simulink model "DQN_ABC_Test"  (R2023b)
settings: Solver=ode23tb  StartTime=0.0  StopTime=0.1  FixedStep=Ts  RelTol=1e-3
values from neighbouring files (symbols this model uses):
  Carm = 3.76    [DQn_ABC_Test_calc.m]
  L = Ld + Lm    [DQn_ABC_Test_calc.m]
  La = 1e-3    (= 0.001)    [DQn_ABC_Test_calc.m]
  Lb = 2*La    (= 0.002)    [DQn_ABC_Test_calc.m]
  Lc = 0.5*La    (= 0.0005)    [DQn_ABC_Test_calc.m]
  N = 1    [DQn_ABC_Test_calc.m]
  R = Rd + Rm    [DQn_ABC_Test_calc.m]
  Ra = 1.64    [DQn_ABC_Test_calc.m]
  Rb = 1.4*Ra    (= 2.296)    [DQn_ABC_Test_calc.m]
  Rc = 2.8*Ra    (= 4.592)    [DQn_ABC_Test_calc.m]
  Ta_dqn = oDP.Ta_dqn    [DQn_ABC_Test_calc.m]
  Ts = 50e-6    (= 5e-05)    [DQn_ABC_Test_calc.m]
  Ts_dqn = Ts    (= 5e-05)    [DQn_ABC_Test_calc.m]
  Ts_emt = Ts    (= 5e-05)    [DQn_ABC_Test_calc.m]
  Ws = 2*pi*f    (= 314.159265359)    [DQn_ABC_Test_calc.m]
undefined symbols (not defined in the file or in its folder): DiscIntNeverNeededParam, i, Xdcpnz, Xdcpnz_c, Xpnz, Ydcpnz, Ydcpnz_c, Ypnz
libraries: DQN_Lib x81, spsCurrentMeasurementLib x9, spsControlledVoltageSourceLib x9, spsSeriesRLCBranchLib x6, spsGroundLib x6, simulink x3, spsMutualInductanceLib x1, spspowerguiLib x1
(part 3 of 6)

== matlab function DQN_ABC_Test/Mult_DQN_Mat4 ==
  data: Xdcpnz_c input; Ydcpnz_c input; Z_DQN output; N parameter; HrmDbl parameter; Zdcpnz_c output
function [Z_DQN, Zdcpnz_c]   = MultDQN(Xdcpnz_c, Ydcpnz_c, N, HrmDbl)

    X_DQN = zeros(N+1,6);
    Y_DQN = zeros(N+1,6);
    Z_DQN = zeros(2*N+1,6);
    Zdcpnz_c = complex(zeros(3,2*N+1));

    X_DQN(1,4) =  2*real(Xdcpnz_c(1,1));
    X_DQN(1,5) =  2*real(Xdcpnz_c(2,1));
    X_DQN(1,6) =  real(Xdcpnz_c(3,1));

    X_DQN(1,1) =  -2*imag(Xdcpnz_c(1,1));
    X_DQN(1,2) =  2*imag(Xdcpnz_c(2,1));
    X_DQN(1,3) =  imag(Xdcpnz_c(3,1));

    Y_DQN(1,4) =  2*real(Ydcpnz_c(1,1));
    Y_DQN(1,5) =  2*real(Ydcpnz_c(2,1));
    Y_DQN(1,6) =  real(Ydcpnz_c(3,1));

    Y_DQN(1,1) =  -2*imag(Ydcpnz_c(1,1));
    Y_DQN(1,2) =  2*imag(Ydcpnz_c(2,1));
    Y_DQN(1,3) =  imag(Ydcpnz_c(3,1));
    
    for i = 2 : N + 1
    
        X_DQN(i,1) =  real(Xdcpnz_c(1,i));
        X_DQN(i,2) = -real(Xdcpnz_c(2,i));
        X_DQN(i,3) =  real(Xdcpnz_c(3,i));

        X_DQN(i,4) =  imag(Xdcpnz_c(1,i));
        X_DQN(i,5) =  imag(Xdcpnz_c(2,i));
        X_DQN(i,6) =  imag(Xdcpnz_c(3,i));

        Y_DQN(i,1) =  real(Ydcpnz_c(1,i));
        Y_DQN(i,2) = -real(Ydcpnz_c(2,i));
        Y_DQN(i,3) =  real(Ydcpnz_c(3,i));

        Y_DQN(i,4) =  imag(Ydcpnz_c(1,i));
        Y_DQN(i,5) =  imag(Ydcpnz_c(2,i));
        Y_DQN(i,6) =  imag(Ydcpnz_c(3,i));
    
    end


%%%%%%%%%%%%%%%%%%%%%%%%%%%%%%

    Xdp = X_DQN(:,1);
    Xdn = X_DQN(:,2);
    Xdz = X_DQN(:,3);
    Xqp = X_DQN(:,4);
    Xqn = X_DQN(:,5);
    Xqz = X_DQN(:,6);
    
    Ydp = Y_DQN(:,1);
    Ydn = Y_DQN(:,2);
    Ydz = Y_DQN(:,3);
    Yqp = Y_DQN(:,4);
    Yqn = Y_DQN(:,5);
    Yqz = Y_DQN(:,6);
    
    Xdc = zeros(6,1);
    Ydc = zeros(6,1);
    Zdc = zeros(6,1);

    Xdc(1) = Xdp(1);
    Xdc(2) = Xdn(1);
    Xdc(3) = Xdz(1);
    Xdc(4) = Xqp(1);
    Xdc(5) = Xqn(1);
    Xdc(6) = Xqz(1);

    Ydc(1) = Ydp(1);
    Ydc(2) = Ydn(1);
    Ydc(3) = Ydz(1);
    Ydc(4) = Yqp(1);
    Ydc(5) = Yqn(1);
    Ydc(6) = Yqz(1);

    a = -0.5+0.866i;
    a2 = -0.5-0.866i;
    T = [1 1 1;1 a a2;1 a2 a];    

    Xdp = [Xdp(2:end); zeros(N-numel(Xdp)+1,1)];
    Ydp = [Ydp(2:end); zeros(N-numel(Ydp)+1,1)];
    Xqp = [Xqp(2:end); zeros(N-numel(Xqp)+1,1)];
    Yqp = [Yqp(2:end); zeros(N-numel(Yqp)+1,1)];
      
    Xdn = [Xdn(2:end); zeros(N-numel(Xdn)+1,1)];
    Ydn = [Ydn(2:end); zeros(N-numel(Ydn)+1,1)];
    Xqn = [Xqn(2:end); zeros(N-numel(Xqn)+1,1)];
    Yqn = [Yqn(2:end); zeros(N-numel(Yqn)+1,1)];
    
    Xdz = [Xdz(2:end); zeros(N-numel(Xdz)+1,1)];
    Ydz = [Ydz(2:end); zeros(N-numel(Ydz)+1,1)];
    Xqz = [Xqz(2:end); zeros(N-numel(Xqz)+1,1)];
    Yqz = [Yqz(2:end); zeros(N-numel(Yqz)+1,1)];
    
   

    Tad_p = [0      -sqrt(1/3)   sqrt(1/3);
            (2/3)   -(1/3)      -(1/3);
            (1/3)    (1/3)       (1/3)];

    Tda_p = [-0           1     1;
             -sqrt(3/4)  -0.5   1;
              sqrt(3/4)  -0.5   1;];


    Tdqn_a = [Tda_p(:,1)  Tda_p(:,1)  0*Tda_p(:,3)  Tda_p(:,2)  Tda_p(:,2)  2*Tda_p(:,3)]/2;
    Ta_dqn = [Tad_p(1,:); Tad_p(1,:); 0*Tad_p(3,:); Tad_p(2,:); Tad_p(2,:); Tad_p(3,:)];
    
    if(0)

        Zdc([1,4, 3]) = Tad_p*((Tda_p*Xdc([1,4,3])).*(Tda_p*Ydc([1,4,3])));
    
    else

        a = -0.5+0.866i;
        a2 = -0.5-0.866i;
        Sas = [1,a,a2;1,a2,a;1,1,1]/3;
        Ssa = inv(Sas);
       

        Zdc = Ta_dqn*((Tdqn_a*Xdc).*(Tdqn_a*Ydc));

    end
    
         
    %Zdc = Xdc.*Ydc;
       
    for h = 1 : 2*N
        if(h<=N)

            Zdc = Zdc + Ta_dqn*0.5*((Xdp(h)*Ydp(h)+Xqp(h)*Yqp(h)+Xdn(h)*Ydn(h)+Xqn(h)*Yqn(h)+Xdz(h)*Ydz(h)+Xqz(h)*Yqz(h))*[1;1;1]);

            %Zdc = Zdc + 0.5*real(Xdcpnz_c(:,h)'*Ydcpnz_c(:,h))*[0;0;0;0;0;-1/3];

            Ymp = sqrt(Ydp(h)^2+Yqp(h)^2);
            Yap = atan2(Yqp(h),+Ydp(h));  


            Ymn = sqrt(Ydn(h)^2+Yqn(h)^2);
            Yan = atan2(Yqn(h),-Ydn(h));  

            Xmz = sqrt(Xdz(h)^2+Xqz(h)^2);
            Xaz = atan2(Xqz(h),+Xdz(h));  
            Ymz = sqrt(Ydz(h)^2+Yqz(h)^2);
            Yaz = atan2(Yqz(h),+Ydz(h));  

            
            Xmp = sqrt(Xdp(h)^2+Xqp(h)^2);
            Xap = atan2(Xqp(h),+Xdp(h));  

            if(Xmp~=0)
                Z_DQN(2*h+1,3) = Z_DQN(2*h+1,3) + 0.5*Xmp*Ymn*sin(Xap+Yan);
                Z_DQN(2*h+1,6) = Z_DQN(2*h+1,6) - 0.5*Xmp*Ymn*cos(Xap+Yan);
    
                Zdc = Zdc + Ta_dqn*0.5*Xmp*Ymn*[cos(Xap-Yan); cos(Xap-Yan-4*pi/3); cos(Xap-Yan+4*pi/3)];
                Zdc = Zdc + Ta_dqn*0.5*Xmp*Ymz*[cos(Xap-Yaz); cos(Xap-Yaz+4*pi/3); cos(Xap-Yaz-4*pi/3)];
            end

            Xmn = sqrt(Xdn(h)^2+Xqn(h)^2);
            Xan = atan2(Xqn(h),-Xdn(h));  

            if(Xmn~=0)
                Z_DQN(2*h+1,3) = Z_DQN(2*h+1,3) + 0.5*Xmn*Ymp*sin(Xan+Yap);
                Z_DQN(2*h+1,6) = Z_DQN(2*h+1,6) - 0.5*Xmn*Ymp*cos(Xan+Yap);
    
                Zdc = Zdc + Ta_dqn*0.5*Xmn*Ymp*[cos(Xan-Yap); cos(Xan-Yap+4*pi/3); cos(Xan-Yap-4*pi/3)];
                Zdc = Zdc + Ta_dqn*0.5*Xmn*Ymz*[cos(Xan-Yaz); cos(Xan-Yaz-4*pi/3); cos(Xan-Yaz+4*pi/3)];
            end
            
            if(Xmz~=0)

                Zdc = Zdc + Ta_dqn*0.5*Xmz*Ymp*[cos(Xaz-Yap); cos(Xaz-Yap-4*pi/3); cos(Xaz-Yap+4*pi/3)];
                Zdc = Zdc + Ta_dqn*0.5*Xmz*Ymn*[cos(Xaz-Yan); cos(Xaz-Yan+4*pi/3); cos(Xaz-Yan-4*pi/3)];

            end

            if(all(Xdc == Xdc(1)) && all(Ydc == Ydc(1)))
                Z_DQN(h+1,1) = Z_DQN(h+1,1)+ Xdc(1)*Ydp(h)+Xdp(h)*Ydc(1);     
                Z_DQN(h+1,4) = Z_DQN(h+1,4)+ Xdc(1)*Yqp(h)+Xqp(h)*Ydc(1);  
                Z_DQN(h+1,2) = Z_DQN(h+1,2)+ Xdc(1)*Ydn(h)+Xdn(h)*Ydc(1);
                Z_DQN(h+1,5) = Z_DQN(h+1,5)+ Xdc(1)*Yqn(h)+Xqn(h)*Ydc(1);
                Z_DQN(h+1,3) = Z_DQN(h+1,3)+ Xdc(1)*Ydz(h)+Xdz(h)*Ydc(1);     
                Z_DQN(h+1,6) = Z_DQN(h+1,6) + Xdc(1)*Yqz(h)+Xqz(h)*Ydc(1); 
            else
                %%%%%%%%%%%%%%%%% POSITIVE (Ydc*Xp) %%%%%%%%%%%%%%%%%%%
                if(Xmp ~= 0)
                    %Y_abc = Tda_p*Ydc([1,4,3]); 
                    Y_abc = Tdqn_a*Ydc; 
                    V_012 = T*[Y_abc(1)*Xmp*(cos(Xap)       +1i*sin(Xap));
                               Y_abc(2)*Xmp*(cos(Xap-2*pi/3)+1i*sin(Xap-2*pi/3));
                               Y_abc(3)*Xmp*(cos(Xap+2*pi/3)+1i*sin(Xap+2*pi/3))]/3;

                    Z_DQN(h+1,3)= Z_DQN(h+1,3)+ real(V_012(1)); Z_DQN(h+1,6) = Z_DQN(h+1,6) + imag(V_012(1));
                    Z_DQN(h+1,1)= Z_DQN(h+1,1)+ real(V_012(2)); Z_DQN(h+1,4)= Z_DQN(h+1,4)+ imag(V_012(2));
                    Z_DQN(h+1,2)= Z_DQN(h+1,2)- real(V_012(3)); Z_DQN(h+1,5)= Z_DQN(h+1,5)+ imag(V_012(3));
                end
                %%%%%%%%%%%%%%%%% POSITIVE (Xdc*Yp) %%%%%%%%%%%%%%%%%%%
                if(Ymp ~= 0)
                    %X_abc = Tda_p*Xdc([1,4,3]); 
                    X_abc = Tdqn_a*Xdc; 
                    V_012 = T*[X_abc(1)*Ymp*(cos(Yap)       +1i*sin(Yap));
                               X_abc(2)*Ymp*(cos(Yap-2*pi/3)+1i*sin(Yap-2*pi/3));
                               X_abc(3)*Ymp*(cos(Yap+2*pi/3)+1i*sin(Yap+2*pi/3))]/3;

                    Z_DQN(h+1,3)= Z_DQN(h+1,3)+ real(V_012(1)); Z_DQN(h+1,6) = Z_DQN(h+1,6) + imag(V_012(1));
                    Z_DQN(h+1,1)= Z_DQN(h+1,1)+ real(V_012(2)); Z_DQN(h+1,4)= Z_DQN(h+1,4)+ imag(V_012(2));
                    Z_DQN(h+1,2)= Z_DQN(h+1,2)- real(V_012(3)); Z_DQN(h+1,5)= Z_DQN(h+1,5)+ imag(V_012(3));
                end
                %%%%%%%%%%%%%%%%% NEGATIVE (Ydc*Xn) %%%%%%%%%%%%%%%%%%%
                if(Xmn ~= 0)
                    %Y_abc = Tda_p*Ydc([1,4,3]); 
                    Y_abc = Tdqn_a*Ydc; 
                    V_012 = T*[Y_abc(1)*Xmn*(cos(Xan)       +1i*sin(Xan));
                               Y_abc(2)*Xmn*(cos(Xan+2*pi/3)+1i*sin(Xan+2*pi/3));
                               Y_abc(3)*Xmn*(cos(Xan-2*pi/3)+1i*sin(Xan-2*pi/3))]/3;
                    

                    Z_DQN(h+1,3)= Z_DQN(h+1,3)+ real(V_012(1)); Z_DQN(h+1,6) = Z_DQN(h+1,6) + imag(V_012(1));
                    Z_DQN(h+1,1)= Z_DQN(h+1,1)+ real(V_012(2)); Z_DQN(h+1,4)= Z_DQN(h+1,4)+ imag(V_012(2));
                    Z_DQN(h+1,2)= Z_DQN(h+1,2)- real(V_012(3)); Z_DQN(h+1,5)= Z_DQN(h+1,5)+ imag(V_012(3));
                end
                %%%%%%%%%%%%%%%%% NEGATIVE (Xdc*Yn) %%%%%%%%%%%%%%%%%%%
                if(Ymn ~= 0)
                    %X_abc = Tda_p*Xdc([1,4,3]); 
                    X_abc = Tdqn_a*Xdc; 
                    V_012 = T*[X_abc(1)*Ymn*(cos(Yan)       +1i*sin(Yan));
                               X_abc(2)*Ymn*(cos(Yan+2*pi/3)+1i*sin(Yan+2*pi/3));
                               X_abc(3)*Ymn*(cos(Yan-2*pi/3)+1i*sin(Yan-2*pi/3))]/3;

                    Z_DQN(h+1,3)= Z_DQN(h+1,3)+ real(V_012(1)); Z_DQN(h+1,6) = Z_DQN(h+1,6) + imag(V_012(1));
                    Z_DQN(h+1,1)= Z_DQN(h+1,1)+ real(V_012(2)); Z_DQN(h+1,4)= Z_DQN(h+1,4)+ imag(V_012(2));
                    Z_DQN(h+1,2)= Z_DQN(h+1,2)- real(V_012(3)); Z_DQN(h+1,5)= Z_DQN(h+1,5)+ imag(V_012(3));
                end
                %%%%%%%%%%%%%%%%%%%%%%%%%%%%%%%%%%%%%%%%%%%%%%%%%%%%%%
                if(Xmz ~= 0)
                    %Y_abc = Tda_p*Ydc([1,4,3]); 
                    Y_abc = Tdqn_a*Ydc; 
                    V_012 = T*[Y_abc(1)*Xmz*(cos(Xaz)+1i*sin(Xaz));
                               Y_abc(2)*Xmz*(cos(Xaz)+1i*sin(Xaz));
                               Y_abc(3)*Xmz*(cos(Xaz)+1i*sin(Xaz))]/3;
                    
                    Z_DQN(h+1,3)= Z_DQN(h+1,3)+ real(V_012(1)); Z_DQN(h+1,6) = Z_DQN(h+1,6) + imag(V_012(1));
                    Z_DQN(h+1,1)= Z_DQN(h+1,1)+ real(V_012(2)); Z_DQN(h+1,4)= Z_DQN(h+1,4)+ imag(V_012(2));
                    Z_DQN(h+1,2)= Z_DQN(h+1,2)- real(V_012(3)); Z_DQN(h+1,5)= Z_DQN(h+1,5)+ imag(V_012(3));
                end
                %%%%%%%%%%%%%%%%%%%%%%%%%%%%%%%%%%%%%%%%%%%%%%%%%%%%%%

                if(Ymz ~= 0)
                    %X_abc = Tda_p*Xdc([1,4,3]); 
                    X_abc = Tdqn_a*Xdc; 
                    V_012 = T*[X_abc(1)*Ymz*(cos(Yaz)+1i*sin(Yaz));
                               X_abc(2)*Ymz*(cos(Yaz)+1i*sin(Yaz));
                               X_abc(3)*Ymz*(cos(Yaz)+1i*sin(Yaz))]/3;
                    
                    Z_DQN(h+1,3)= Z_DQN(h+1,3)+ real(V_012(1)); Z_DQN(h+1,6) = Z_DQN(h+1,6) + imag(V_012(1));
                    Z_DQN(h+1,1)= Z_DQN(h+1,1)+ real(V_012(2)); Z_DQN(h+1,4)= Z_DQN(h+1,4)+ imag(V_012(2));
                    Z_DQN(h+1,2)= Z_DQN(h+1,2)- real(V_012(3)); Z_DQN(h+1,5)= Z_DQN(h+1,5)+ imag(V_012(3));
                end
            end
            
%%%%%%%%%%%%%%%%%%%%%% h<=N ODD %%%%%%%%%%%%%%%%%%%%%%%%%%%%%%%%%%%%%%%%%
            if(mod(h,2)==1) 
                %%%%%%%%%%%%%%%%% D3p (3ph+) %%%%%%%%%%%%%%%%%%%%%%%

                %&%%%%%%%%%%%%%%%%%%%%%%%%%% PP + NN %%%%%%%%%%%%%%%%%%%%%%%%%%%
                for i = 1 : h - 1
                   Z_DQN(h+1,1)= Z_DQN(h+1,1)- 0.5*(Xdn(i)*Yqn(h-i) + Xqn(i)*Ydn(h-i));                    
                   Z_DQN(h+1,2)= Z_DQN(h+1,2)- 0.5*(Xdp(i)*Yqp(h-i) + Xqp(i)*Ydp(h-i)); 
                   Z_DQN(h+1,4)= Z_DQN(h+1,4)- 0.5*(Xdn(i)*Ydn(h-i) - Xqn(i)*Yqn(h-i));                
                   Z_DQN(h+1,5)= Z_DQN(h+1,5)- 0.5*(Xdp(i)*Ydp(h-i) - Xqp(i)*Yqp(h-i)); 
                end

                for i = 1 : N - h
                    Z_DQN(h+1,3)= Z_DQN(h+1,3)+ 0.5*(-Xdp(i)*Yqp(i+h) + Xqp(i)*Ydp(i+h) + Xdp(i+h)*Yqp(i) - Xqp(i+h)*Ydp(i) + Xdn(i)*Yqn(i+h) - Xqn(i)*Ydn(i+h) - Xdn(i+h)*Yqn(i) + Xqn(i+h)*Ydn(i));  
                    Z_DQN(h+1,6) = Z_DQN(h+1,6) + 0.5*(+Xdp(i)*Ydp(i+h) + Xqp(i)*Yqp(i+h) + Xdp(i+h)*Ydp(i) + Xqp(i+h)*Yqp(i) + Xdn(i)*Ydn(i+h) + Xqn(i)*Yqn(i+h) + Xdn(i+h)*Ydn(i) + Xqn(i+h)*Yqn(i));    
                end
                %&%%%%%%%%%%%%%%%%%%%%%%%%%% PP + NN %%%%%%%%%%%%%%%%%%%%%%%%%%%

                for k = 1 : (N + mod(N+1,2) - h)/2
                    i = 2*k-1;
                    j = i+h;

                    Z_DQN(h+1,3) = Z_DQN(h+1,3) + 0.5*(-Xdz(i)*Yqz(j) + Xqz(i)*Ydz(j) + Xdz(j)*Yqz(i) - Xqz(j)*Ydz(i));
                    Z_DQN(h+1,6)  = Z_DQN(h+1,6)  + 0.5*(+Xdz(i)*Ydz(j) + Xqz(i)*Yqz(j) + Xdz(j)*Ydz(i) + Xqz(j)*Yqz(i)); 

                    Z_DQN(h+1,1)= Z_DQN(h+1,1)+ 0.5*(-Xdp(i)*Yqn(j) - Xqp(i)*Ydn(j) - Xdn(j)*Yqp(i) - Xqn(j)*Ydp(i)); 
                    Z_DQN(h+1,1)= Z_DQN(h+1,1)+ 0.5*(-Xdz(i)*Yqp(j) + Xqz(i)*Ydp(j) + Xdp(j)*Yqz(i) - Xqp(j)*Ydz(i));    
                    Z_DQN(h+1,1)= Z_DQN(h+1,1)+ 0.5*(+Xdn(i)*Yqz(j) + Xqn(i)*Ydz(j) + Xdz(j)*Yqn(i) + Xqz(j)*Ydn(i));
                    
                    Z_DQN(h+1,4)= Z_DQN(h+1,4)+ 0.5*(-Xdp(i)*Ydn(j) + Xqp(i)*Yqn(j) - Xdn(j)*Ydp(i) + Xqn(j)*Yqp(i));  
                    Z_DQN(h+1,4)= Z_DQN(h+1,4)+ 0.5*(+Xdz(i)*Ydp(j) + Xqz(i)*Yqp(j) + Xdp(j)*Ydz(i) + Xqp(j)*Yqz(i));     
                    Z_DQN(h+1,4)= Z_DQN(h+1,4)+ 0.5*(-Xdn(i)*Ydz(j) + Xqn(i)*Yqz(j) - Xdz(j)*Ydn(i) + Xqz(j)*Yqn(i));

                    Z_DQN(h+1,2)= Z_DQN(h+1,2)+ 0.5*(+Xdp(i)*Yqz(j) - Xqp(i)*Ydz(j) - Xdz(j)*Yqp(i) + Xqz(j)*Ydp(i));             
                    Z_DQN(h+1,2)= Z_DQN(h+1,2)+ 0.5*(+Xdz(i)*Yqn(j) + Xqz(i)*Ydn(j) + Xdn(j)*Yqz(i) + Xqn(j)*Ydz(i));
                    Z_DQN(h+1,2)= Z_DQN(h+1,2)+ 0.5*(-Xdn(i)*Yqp(j) - Xqn(i)*Ydp(j) - Xdp(j)*Yqn(i) - Xqp(j)*Ydn(i)); 

                    Z_DQN(h+1,5)= Z_DQN(h+1,5)+ 0.5*(+Xdp(i)*Ydz(j) + Xqp(i)*Yqz(j) + Xdz(j)*Ydp(i) + Xqz(j)*Yqp(i)); 
                    Z_DQN(h+1,5)= Z_DQN(h+1,5)+ 0.5*(-Xdz(i)*Ydn(j) + Xqz(i)*Yqn(j) - Xdn(j)*Ydz(i) + Xqn(j)*Yqz(i)); 
                    Z_DQN(h+1,5)= Z_DQN(h+1,5)+ 0.5*(-Xdn(i)*Ydp(j) + Xqn(i)*Yqp(j) - Xdp(j)*Ydn(i) + Xqp(j)*Yqn(i));  
                end

                for k = 1 : (N + mod(N,2) - h - 1)/2
                    i = 2*k;
                    j = i+h;
                    
                    Z_DQN(h+1,3)= Z_DQN(h+1,3)  + 0.5*(-Xdz(i)*Yqz(j) + Xqz(i)*Ydz(j) + Xdz(j)*Yqz(i) - Xqz(j)*Ydz(i));
                    Z_DQN(h+1,6) = Z_DQN(h+1,6)   + 0.5*(+Xdz(i)*Ydz(j) + Xqz(i)*Yqz(j) + Xdz(j)*Ydz(i) + Xqz(j)*Yqz(i)); 

                    Z_DQN(h+1,1)= Z_DQN(h+1,1)+ 0.5*(-Xdp(i)*Yqn(j) - Xqp(i)*Ydn(j) - Xdn(j)*Yqp(i) - Xqn(j)*Ydp(i)); 
                    Z_DQN(h+1,4)= Z_DQN(h+1,4)+ 0.5*(-Xdp(i)*Ydn(j) + Xqp(i)*Yqn(j) - Xdn(j)*Ydp(i) + Xqn(j)*Yqp(i));  
                    Z_DQN(h+1,2)= Z_DQN(h+1,2)+ 0.5*(-Xdn(i)*Yqp(j) - Xqn(i)*Ydp(j) - Xdp(j)*Yqn(i) - Xqp(j)*Ydn(i)); 
                    Z_DQN(h+1,5)= Z_DQN(h+1,5)+ 0.5*(-Xdn(i)*Ydp(j) + Xqn(i)*Yqp(j) - Xdp(j)*Ydn(i) + Xqp(j)*Yqn(i));                                          

                    Z_DQN(h+1,1)= Z_DQN(h+1,1)+ 0.5*(-Xdz(i)*Yqp(j) + Xqz(i)*Ydp(j) + Xdp(j)*Yqz(i) - Xqp(j)*Ydz(i));
                    Z_DQN(h+1,4)= Z_DQN(h+1,4)+ 0.5*(+Xdz(i)*Ydp(j) + Xqz(i)*Yqp(j) + Xdp(j)*Ydz(i) + Xqp(j)*Yqz(i));                     
                    Z_DQN(h+1,2)= Z_DQN(h+1,2)+ 0.5*(+Xdp(i)*Yqz(j) - Xqp(i)*Ydz(j) - Xdz(j)*Yqp(i) + Xqz(j)*Ydp(i));
                    Z_DQN(h+1,5)= Z_DQN(h+1,5)+ 0.5*(+Xdp(i)*Ydz(j) + Xqp(i)*Yqz(j) + Xdz(j)*Ydp(i) + Xqz(j)*Yqp(i));   

                    Z_DQN(h+1,1)= Z_DQN(h+1,1)+ 0.5*(+Xdn(i)*Yqz(j) + Xqn(i)*Ydz(j) + Xdz(j)*Yqn(i) + Xqz(j)*Ydn(i));
                    Z_DQN(h+1,4)= Z_DQN(h+1,4)+ 0.5*(-Xdn(i)*Ydz(j) + Xqn(i)*Yqz(j) - Xdz(j)*Ydn(i) + Xqz(j)*Yqn(i));                
                    Z_DQN(h+1,2)= Z_DQN(h+1,2)+ 0.5*(+Xdz(i)*Yqn(j) + Xqz(i)*Ydn(j) + Xdn(j)*Yqz(i) + Xqn(j)*Ydz(i));
                    Z_DQN(h+1,5)= Z_DQN(h+1,5)+ 0.5*(-Xdz(i)*Ydn(j) + Xqz(i)*Yqn(j) - Xdn(j)*Ydz(i) + Xqn(j)*Yqz(i)); 

                end

                for k = (h-1)/2:-1:1
                    i = k;
                    j = h-i;  
                    
                    Z_DQN(h+1,3)= Z_DQN(h+1,3)+ 0.5*(+Xdp(i)*Yqn(j)-Xqp(i)*Ydn(j)-Xdn(j)*Yqp(i)+Xqn(j)*Ydp(i));
                    Z_DQN(h+1,6) = Z_DQN(h+1,6) + 0.5*(+Xdp(i)*Ydn(j)+Xqp(i)*Yqn(j)+Xdn(j)*Ydp(i)+Xqn(j)*Yqp(i));
                    Z_DQN(h+1,3)= Z_DQN(h+1,3)+ 0.5*(+Xdp(j)*Yqn(i)-Xqp(j)*Ydn(i)-Xdn(i)*Yqp(j)+Xqn(i)*Ydp(j));
                    Z_DQN(h+1,6) = Z_DQN(h+1,6) + 0.5*(+Xdp(j)*Ydn(i)+Xqp(j)*Yqn(i)+Xdn(i)*Ydp(j)+Xqn(i)*Yqp(j)); 
                    Z_DQN(h+1,3)= Z_DQN(h+1,3)+ 0.5*(+Xdz(i)*Yqz(j)+Xqz(i)*Ydz(j)+Xdz(j)*Yqz(i)+Xqz(j)*Ydz(i));
                    Z_DQN(h+1,6) = Z_DQN(h+1,6) + 0.5*(-Xdz(i)*Ydz(j)+Xqz(i)*Yqz(j)-Xdz(j)*Ydz(i)+Xqz(j)*Yqz(i));    
                        
                        
                    Z_DQN(h+1,1)= Z_DQN(h+1,1)+ 0.5*(+Xdz(i)*Yqp(j)+Xqz(i)*Ydp(j)+Xdz(j)*Yqp(i)+Xqz(j)*Ydp(i));
                    Z_DQN(h+1,4)= Z_DQN(h+1,4)+ 0.5*(-Xdz(i)*Ydp(j)+Xqz(i)*Yqp(j)-Xdz(j)*Ydp(i)+Xqz(j)*Yqp(i));
                    Z_DQN(h+1,1)= Z_DQN(h+1,1)+ 0.5*(+Xdp(i)*Yqz(j)+Xqp(i)*Ydz(j)+Xdp(j)*Yqz(i)+Xqp(j)*Ydz(i));
                    Z_DQN(h+1,4)= Z_DQN(h+1,4)+ 0.5*(-Xdp(i)*Ydz(j)+Xqp(i)*Yqz(j)-Xdp(j)*Ydz(i)+Xqp(j)*Yqz(i)); 
                    
                              
                    Z_DQN(h+1,2)= Z_DQN(h+1,2)+ 0.5*(+Xdn(i)*Yqz(j)-Xqn(i)*Ydz(j)+Xdn(j)*Yqz(i)-Xqn(j)*Ydz(i));
                    Z_DQN(h+1,5)= Z_DQN(h+1,5)+ 0.5*(+Xdn(i)*Ydz(j)+Xqn(i)*Yqz(j)+Xdn(j)*Ydz(i)+Xqn(j)*Yqz(i)); 
                    Z_DQN(h+1,2)= Z_DQN(h+1,2)+ 0.5*(-Xdz(i)*Yqn(j)+Xqz(i)*Ydn(j)-Xdz(j)*Yqn(i)+Xqz(j)*Ydn(i));
                    Z_DQN(h+1,5)= Z_DQN(h+1,5)+ 0.5*(+Xdz(i)*Ydn(j)+Xqz(i)*Yqn(j)+Xdz(j)*Ydn(i)+Xqz(j)*Yqn(i)); 
                end
%%%%%%%%%%%%%%%%%%%%%% h<=N EVEN %%%%%%%%%%%%%%%%%%%%%%%%%%%%%%%%%%%%%%%%%           
            else 
               
                Z_DQN(h+1,1)= Z_DQN(h+1,1)+ 0.5*(-Xdn(h/2)*Yqn(h/2)-Xqn(h/2)*Ydn(h/2));   
                Z_DQN(h+1,4)= Z_DQN(h+1,4)+ 0.5*(-Xdn(h/2)*Ydn(h/2)+Xqn(h/2)*Yqn(h/2)); 
                Z_DQN(h+1,2)= Z_DQN(h+1,2)+ 0.5*(-Xdp(h/2)*Yqp(h/2)-Xqp(h/2)*Ydp(h/2));   
                Z_DQN(h+1,5)= Z_DQN(h+1,5)+ 0.5*(-Xdp(h/2)*Ydp(h/2)+Xqp(h/2)*Yqp(h/2));   

                Z_DQN(h+1,3) = Z_DQN(h+1,3) + 0.5*(+Xdz(h/2)*Yqz(h/2)+Xqz(h/2)*Ydz(h/2));
                Z_DQN(h+1,6)  = Z_DQN(h+1,6)  + 0.5*(-Xdz(h/2)*Ydz(h/2)+Xqz(h/2)*Yqz(h/2));

                Z_DQN(h+1,1)= Z_DQN(h+1,1)+ 0.5*(+Xdz(h/2)*Yqp(h/2)+Xqz(h/2)*Ydp(h/2)+Xdp(h/2)*Yqz(h/2)+Xqp(h/2)*Ydz(h/2));   
                Z_DQN(h+1,4)= Z_DQN(h+1,4)+ 0.5*(-Xdz(h/2)*Ydp(h/2)+Xqz(h/2)*Yqp(h/2)-Xdp(h/2)*Ydz(h/2)+Xqp(h/2)*Yqz(h/2)); 
                Z_DQN(h+1,2)= Z_DQN(h+1,2)+ 0.5*(+Xdn(h/2)*Yqz(h/2)-Xqn(h/2)*Ydz(h/2)-Xdz(h/2)*Yqn(h/2)+Xqz(h/2)*Ydn(h/2));   
                Z_DQN(h+1,5)= Z_DQN(h+1,5)+ 0.5*(+Xdn(h/2)*Ydz(h/2)+Xqn(h/2)*Yqz(h/2)+Xdz(h/2)*Ydn(h/2)+Xqz(h/2)*Yqn(h/2));    
                
                for k = 1:N-h
                    i = k;
                    j = h+i;
                
                    Z_DQN(h+1,3)= Z_DQN(h+1,3)  + 0.5*(+Xdp(j)*Yqp(i) - Xqp(j)*Ydp(i) - Xdp(i)*Yqp(j) + Xqp(i)*Ydp(j));
                    Z_DQN(h+1,6) = Z_DQN(h+1,6)   + 0.5*(+Xdp(j)*Ydp(i) + Xqp(j)*Yqp(i) + Xdp(i)*Ydp(j) + Xqp(i)*Yqp(j));                                           
                    Z_DQN(h+1,3)= Z_DQN(h+1,3)  + 0.5*(+Xdn(i)*Yqn(j) - Xqn(i)*Ydn(j) - Xdn(j)*Yqn(i) + Xqn(j)*Ydn(i));
                    Z_DQN(h+1,6) = Z_DQN(h+1,6)   + 0.5*(+Xdn(i)*Ydn(j) + Xqn(i)*Yqn(j) + Xdn(j)*Ydn(i) + Xqn(j)*Yqn(i));  
                    Z_DQN(h+1,3)= Z_DQN(h+1,3)  + 0.5*(-Xdz(i)*Yqz(j) + Xqz(i)*Ydz(j) + Xdz(j)*Yqz(i) - Xqz(j)*Ydz(i));
                    Z_DQN(h+1,6) = Z_DQN(h+1,6)   + 0.5*(+Xdz(i)*Ydz(j) + Xqz(i)*Yqz(j) + Xdz(j)*Ydz(i) + Xqz(j)*Yqz(i)); 
                                       
                    Z_DQN(h+1,1)= Z_DQN(h+1,1)+ 0.5*(-Xdp(i)*Yqn(j) - Xqp(i)*Ydn(j) - Xdn(j)*Yqp(i) - Xqn(j)*Ydp(i)); 
                    Z_DQN(h+1,4)= Z_DQN(h+1,4)+ 0.5*(-Xdp(i)*Ydn(j) + Xqp(i)*Yqn(j) - Xdn(j)*Ydp(i) + Xqn(j)*Yqp(i)); 
                    Z_DQN(h+1,2)= Z_DQN(h+1,2)+ 0.5*(-Xdn(i)*Yqp(j) - Xqn(i)*Ydp(j) - Xdp(j)*Yqn(i) - Xqp(j)*Ydn(i)); 
                    Z_DQN(h+1,5)= Z_DQN(h+1,5)+ 0.5*(-Xdn(i)*Ydp(j) + Xqn(i)*Yqp(j) - Xdp(j)*Ydn(i) + Xqp(j)*Yqn(i)); 
                        
                    Z_DQN(h+1,1)= Z_DQN(h+1,1)+ 0.5*(+Xdp(j)*Yqz(i) - Xqp(j)*Ydz(i) - Xdz(i)*Yqp(j) + Xqz(i)*Ydp(j));
                    Z_DQN(h+1,4)= Z_DQN(h+1,4)+ 0.5*(+Xdp(j)*Ydz(i) + Xqp(j)*Yqz(i) + Xdz(i)*Ydp(j) + Xqz(i)*Yqp(j)); 
                    Z_DQN(h+1,2)= Z_DQN(h+1,2)+ 0.5*(+Xdp(i)*Yqz(j) - Xqp(i)*Ydz(j) - Xdz(j)*Yqp(i) + Xqz(j)*Ydp(i));
                    Z_DQN(h+1,5)= Z_DQN(h+1,5)+ 0.5*(+Xdp(i)*Ydz(j) + Xqp(i)*Yqz(j) + Xdz(j)*Ydp(i) + Xqz(j)*Yqp(i)); 
                    
                    Z_DQN(h+1,1)= Z_DQN(h+1,1)+ 0.5*(+Xdn(i)*Yqz(j) + Xqn(i)*Ydz(j) + Xdz(j)*Yqn(i) + Xqz(j)*Ydn(i));
                    Z_DQN(h+1,4)= Z_DQN(h+1,4)+ 0.5*(-Xdn(i)*Ydz(j) + Xqn(i)*Yqz(j) - Xdz(j)*Ydn(i) + Xqz(j)*Yqn(i)); 
                    Z_DQN(h+1,2)= Z_DQN(h+1,2)+ 0.5*(+Xdn(j)*Yqz(i) + Xqn(j)*Ydz(i) + Xdz(i)*Yqn(j) + Xqz(i)*Ydn(j));
                    Z_DQN(h+1,5)= Z_DQN(h+1,5)+ 0.5*(-Xdn(j)*Ydz(i) + Xqn(j)*Yqz(i) - Xdz(i)*Ydn(j) + Xqz(i)*Yqn(j)); 
                end

                for k = h/2-1:-1:1
                    i = k;
                    j = h-i;   

                    Z_DQN(h+1,3)= Z_DQN(h+1,3)  + 0.5*(+Xdp(i)*Yqn(j) - Xqp(i)*Ydn(j) + Xdp(j)*Yqn(i) - Xqp(j)*Ydn(i));
                    Z_DQN(h+1,3)= Z_DQN(h+1,3)  + 0.5*(-Xdn(i)*Yqp(j) + Xqn(i)*Ydp(j) - Xdn(j)*Yqp(i) + Xqn(j)*Ydp(i));      
                    Z_DQN(h+1,3)= Z_DQN(h+1,3)  + 0.5*(+Xdz(i)*Yqz(j) + Xqz(i)*Ydz(j) + Xdz(j)*Yqz(i) + Xqz(j)*Ydz(i));
                    
                    Z_DQN(h+1,6) = Z_DQN(h+1,6)   + 0.5*(+Xdp(i)*Ydn(j) + Xqp(i)*Yqn(j) + Xdp(j)*Ydn(i) + Xqp(j)*Yqn(i)); 
                    Z_DQN(h+1,6) = Z_DQN(h+1,6)   + 0.5*(+Xdn(i)*Ydp(j) + Xqn(i)*Yqp(j) + Xdn(j)*Ydp(i) + Xqn(j)*Yqp(i));
                    Z_DQN(h+1,6) = Z_DQN(h+1,6)   + 0.5*(-Xdz(i)*Ydz(j) + Xqz(i)*Yqz(j) - Xdz(j)*Ydz(i) + Xqz(j)*Yqz(i)); 
                    
                    Z_DQN(h+1,1)= Z_DQN(h+1,1)+ 0.5*(+Xdp(i)*Yqz(j) + Xqp(i)*Ydz(j) + Xdp(j)*Yqz(i) + Xqp(j)*Ydz(i)); 
                    Z_DQN(h+1,1)= Z_DQN(h+1,1)+ 0.5*(-Xdn(i)*Yqn(j) - Xqn(i)*Ydn(j) - Xdn(j)*Yqn(i) - Xqn(j)*Ydn(i)); 
                    Z_DQN(h+1,1)= Z_DQN(h+1,1)+ 0.5*(+Xdz(i)*Yqp(j) + Xqz(i)*Ydp(j) + Xdz(j)*Yqp(i) + Xqz(j)*Ydp(i));
                    
                    Z_DQN(h+1,4)= Z_DQN(h+1,4)+ 0.5*(-Xdp(i)*Ydz(j) + Xqp(i)*Yqz(j) - Xdp(j)*Ydz(i) + Xqp(j)*Yqz(i)); 
                    Z_DQN(h+1,4)= Z_DQN(h+1,4)+ 0.5*(-Xdn(i)*Ydn(j) + Xqn(i)*Yqn(j) - Xdn(j)*Ydn(i) + Xqn(j)*Yqn(i));
                    Z_DQN(h+1,4)= Z_DQN(h+1,4)+ 0.5*(-Xdz(i)*Ydp(j) + Xqz(i)*Yqp(j) - Xdz(j)*Ydp(i) + Xqz(j)*Yqp(i));  
                    
                    Z_DQN(h+1,2)= Z_DQN(h+1,2)+ 0.5*(-Xdp(i)*Yqp(j) - Xqp(i)*Ydp(j) - Xdp(j)*Yqp(i) - Xqp(j)*Ydp(i));
                    Z_DQN(h+1,2)= Z_DQN(h+1,2)+ 0.5*(+Xdn(i)*Yqz(j) - Xqn(i)*Ydz(j) + Xdn(j)*Yqz(i) - Xqn(j)*Ydz(i));
                    Z_DQN(h+1,2)= Z_DQN(h+1,2)+ 0.5*(-Xdz(i)*Yqn(j) + Xqz(i)*Ydn(j) - Xdz(j)*Yqn(i) + Xqz(j)*Ydn(i));
                    
                    Z_DQN(h+1,5)= Z_DQN(h+1,5)+ 0.5*(-Xdp(i)*Ydp(j) + Xqp(i)*Yqp(j) - Xdp(j)*Ydp(i) + Xqp(j)*Yqp(i));  
                    Z_DQN(h+1,5)= Z_DQN(h+1,5)+ 0.5*(+Xdn(i)*Ydz(j) + Xqn(i)*Yqz(j) + Xdn(j)*Ydz(i) + Xqn(j)*Yqz(i));
                    Z_DQN(h+1,5)= Z_DQN(h+1,5)+ 0.5*(+Xdz(i)*Ydn(j) + Xqz(i)*Yqn(j) + Xdz(j)*Ydn(i) + Xqz(j)*Yqn(i)); 
                end
            end
%%%%%%%%%%%%%%%%%%%%%%%%%%%% h>N  %%%%%%%%%%%%%%%%%%%%%%%%%%%%%%%%%%%%%%%%% 
        else %h>N
            if(HrmDbl)
            
                %%%%%%%%%%%%%%%%%%%%%%%%%%% PP + NN %%%%%%%%%%%%%%%%%%%%%%%%%%%
                for i = h-N : N
                    Z_DQN(h+1,1)= Z_DQN(h+1,1)- 0.5*(Xdn(i)*Yqn(h-i) + Xqn(i)*Ydn(h-i));                
                    Z_DQN(h+1,2)= Z_DQN(h+1,2)- 0.5*(Xdp(i)*Yqp(h-i) + Xqp(i)*Ydp(h-i));                     
                    Z_DQN(h+1,4)= Z_DQN(h+1,4)- 0.5*(Xdn(i)*Ydn(h-i) - Xqn(i)*Yqn(h-i));                      
                    Z_DQN(h+1,5)= Z_DQN(h+1,5)- 0.5*(Xdp(i)*Ydp(h-i) - Xqp(i)*Yqp(h-i));   
                end
                %%%%%%%%%%%%%%%%%%%%%%%%%%% PP + NN %%%%%%%%%%%%%%%%%%%%%%%%%%%

                if(mod(h,2)==1) %%%%%%%%%%% h>N ODD %%%%%%%%%%%%%%%%%%%

                    for k = (h-1)/2:-1:h-N
                        i = k;
                        j = h-i;

                        Z_DQN(h+1,3)= Z_DQN(h+1,3)+ 0.5*(+Xdp(i)*Yqn(j)-Xqp(i)*Ydn(j)-Xdn(j)*Yqp(i)+Xqn(j)*Ydp(i));                  
                        Z_DQN(h+1,3)= Z_DQN(h+1,3)+ 0.5*(+Xdp(j)*Yqn(i)-Xqp(j)*Ydn(i)-Xdn(i)*Yqp(j)+Xqn(i)*Ydp(j));
                        Z_DQN(h+1,3)= Z_DQN(h+1,3)+ 0.5*(+Xdz(i)*Yqz(j)+Xqz(i)*Ydz(j)+Xdz(j)*Yqz(i)+Xqz(j)*Ydz(i));

                        Z_DQN(h+1,6) = Z_DQN(h+1,6) + 0.5*(-Xdz(i)*Ydz(j)+Xqz(i)*Yqz(j)-Xdz(j)*Ydz(i)+Xqz(j)*Yqz(i));
                        Z_DQN(h+1,6) = Z_DQN(h+1,6) + 0.5*(+Xdp(i)*Ydn(j)+Xqp(i)*Yqn(j)+Xdn(j)*Ydp(i)+Xqn(j)*Yqp(i));
                        Z_DQN(h+1,6) = Z_DQN(h+1,6) + 0.5*(+Xdp(j)*Ydn(i)+Xqp(j)*Yqn(i)+Xdn(i)*Ydp(j)+Xqn(i)*Yqp(j));  

                        Z_DQN(h+1,1)= Z_DQN(h+1,1)+ 0.5*(+Xdp(i)*Yqz(j)+Xqp(i)*Ydz(j)+Xdp(j)*Yqz(i)+Xqp(j)*Ydz(i));
                        Z_DQN(h+1,1)= Z_DQN(h+1,1)+ 0.5*(+Xdz(i)*Yqp(j)+Xqz(i)*Ydp(j)+Xdz(j)*Yqp(i)+Xqz(j)*Ydp(i));

                        Z_DQN(h+1,4)= Z_DQN(h+1,4)+ 0.5*(-Xdp(i)*Ydz(j)+Xqp(i)*Yqz(j)-Xdp(j)*Ydz(i)+Xqp(j)*Yqz(i)); 
                        Z_DQN(h+1,4)= Z_DQN(h+1,4)+ 0.5*(-Xdz(i)*Ydp(j)+Xqz(i)*Yqp(j)-Xdz(j)*Ydp(i)+Xqz(j)*Yqp(i));     

                        Z_DQN(h+1,2)= Z_DQN(h+1,2)+ 0.5*(+Xdn(i)*Yqz(j)-Xqn(i)*Ydz(j)+Xdn(j)*Yqz(i)-Xqn(j)*Ydz(i));
                        Z_DQN(h+1,2)= Z_DQN(h+1,2)+ 0.5*(-Xdz(i)*Yqn(j)+Xqz(i)*Ydn(j)-Xdz(j)*Yqn(i)+Xqz(j)*Ydn(i));

                        Z_DQN(h+1,5)= Z_DQN(h+1,5)+ 0.5*(+Xdn(i)*Ydz(j)+Xqn(i)*Yqz(j)+Xdn(j)*Ydz(i)+Xqn(j)*Yqz(i));
                        Z_DQN(h+1,5)= Z_DQN(h+1,5)+ 0.5*(+Xdz(i)*Ydn(j)+Xqz(i)*Yqn(j)+Xdz(j)*Ydn(i)+Xqz(j)*Yqn(i));    

                    end

                else %%%%%%%%%%% h>N EVEN %%%%%%%%%%%%%%%%%%%

                    Z_DQN(h+1,3) = Z_DQN(h+1,3) + 0.5*(+Xdz(h/2)*Yqz(h/2)+Xqz(h/2)*Ydz(h/2));
                    Z_DQN(h+1,6)  = Z_DQN(h+1,6)  + 0.5*(-Xdz(h/2)*Ydz(h/2)+Xqz(h/2)*Yqz(h/2));

                    Z_DQN(h+1,1)= 0.5*(-Xdn(h/2)*Yqn(h/2)-Xqn(h/2)*Ydn(h/2));          
                    Z_DQN(h+1,1)= Z_DQN(h+1,1)+ 0.5*(+Xdp(h/2)*Yqz(h/2)+Xqp(h/2)*Ydz(h/2));                
                    Z_DQN(h+1,1)= Z_DQN(h+1,1)+ 0.5*(+Xdz(h/2)*Yqp(h/2)+Xqz(h/2)*Ydp(h/2));    

                    Z_DQN(h+1,4)= 0.5*(-Xdn(h/2)*Ydn(h/2)+Xqn(h/2)*Yqn(h/2));             
                    Z_DQN(h+1,4)= Z_DQN(h+1,4)+ 0.5*(-Xdp(h/2)*Ydz(h/2)+Xqp(h/2)*Yqz(h/2));        
                    Z_DQN(h+1,4)= Z_DQN(h+1,4)+ 0.5*(-Xdz(h/2)*Ydp(h/2)+Xqz(h/2)*Yqp(h/2)); 

                    Z_DQN(h+1,2)= 0.5*(-Xdp(h/2)*Yqp(h/2)-Xqp(h/2)*Ydp(h/2)); 
                    Z_DQN(h+1,2)= Z_DQN(h+1,2)+ 0.5*(+Xdn(h/2)*Yqz(h/2)-Xqn(h/2)*Ydz(h/2));
                    Z_DQN(h+1,2)= Z_DQN(h+1,2)+ 0.5*(-Xdz(h/2)*Yqn(h/2)+Xqz(h/2)*Ydn(h/2));

                    Z_DQN(h+1,5)= 0.5*(-Xdp(h/2)*Ydp(h/2)+Xqp(h/2)*Yqp(h/2)); 
                    Z_DQN(h+1,5)= Z_DQN(h+1,5)+ 0.5*(+Xdn(h/2)*Ydz(h/2)+Xqn(h/2)*Yqz(h/2));        
                    Z_DQN(h+1,5)= Z_DQN(h+1,5)+ 0.5*(+Xdz(h/2)*Ydn(h/2)+Xqz(h/2)*Yqn(h/2)); 

                    for i = (h+2)/2:N
                        j = h-i;
                        Z_DQN(h+1,3) = Z_DQN(h+1,3) + 0.5*(+Xdp(i)*Yqn(j)-Xqp(i)*Ydn(j)+Xdp(j)*Yqn(i)-Xqp(j)*Ydn(i));
                        Z_DQN(h+1,3) = Z_DQN(h+1,3) + 0.5*(-Xdn(i)*Yqp(j)+Xqn(i)*Ydp(j)-Xdn(j)*Yqp(i)+Xqn(j)*Ydp(i));
                        Z_DQN(h+1,3) = Z_DQN(h+1,3) + 0.5*(+Xdz(i)*Yqz(j)+Xqz(i)*Ydz(j)+Xdz(j)*Yqz(i)+Xqz(j)*Ydz(i));

                        Z_DQN(h+1,6)  = Z_DQN(h+1,6)  + 0.5*(+Xdp(i)*Ydn(j)+Xqp(i)*Yqn(j)+Xdp(j)*Ydn(i)+Xqp(j)*Yqn(i));                      
                        Z_DQN(h+1,6)  = Z_DQN(h+1,6)  + 0.5*(+Xdn(i)*Ydp(j)+Xqn(i)*Yqp(j)+Xdn(j)*Ydp(i)+Xqn(j)*Yqp(i));  
                        Z_DQN(h+1,6)  = Z_DQN(h+1,6)  + 0.5*(-Xdz(i)*Ydz(j)+Xqz(i)*Yqz(j)-Xdz(j)*Ydz(i)+Xqz(j)*Yqz(i));

                        Z_DQN(h+1,1)= Z_DQN(h+1,1)+ 0.5*(+Xdp(i)*Yqz(j)+Xqp(i)*Ydz(j)+Xdp(j)*Yqz(i)+Xqp(j)*Ydz(i));  
                        Z_DQN(h+1,1)= Z_DQN(h+1,1)+ 0.5*(-Xdn(i)*Yqn(j)-Xqn(i)*Ydn(j)-Xdn(j)*Yqn(i)-Xqn(j)*Ydn(i));             
                        Z_DQN(h+1,1)= Z_DQN(h+1,1)+ 0.5*(+Xdz(i)*Yqp(j)+Xqz(i)*Ydp(j)+Xdz(j)*Yqp(i)+Xqz(j)*Ydp(i));           

                        Z_DQN(h+1,4)= Z_DQN(h+1,4)+ 0.5*(-Xdp(i)*Ydz(j)+Xqp(i)*Yqz(j)-Xdp(j)*Ydz(i)+Xqp(j)*Yqz(i));
                        Z_DQN(h+1,4)= Z_DQN(h+1,4)+ 0.5*(-Xdn(i)*Ydn(j)+Xqn(i)*Yqn(j)-Xdn(j)*Ydn(i)+Xqn(j)*Yqn(i));    
                        Z_DQN(h+1,4)= Z_DQN(h+1,4)+ 0.5*(-Xdz(i)*Ydp(j)+Xqz(i)*Yqp(j)-Xdz(j)*Ydp(i)+Xqz(j)*Yqp(i));   

                        Z_DQN(h+1,2)= Z_DQN(h+1,2)+ 0.5*(-Xdp(i)*Yqp(j)-Xqp(i)*Ydp(j)-Xdp(j)*Yqp(i)-Xqp(j)*Ydp(i));
                        Z_DQN(h+1,2)= Z_DQN(h+1,2)+ 0.5*(+Xdn(i)*Yqz(j)-Xqn(i)*Ydz(j)+Xdn(j)*Yqz(i)-Xqn(j)*Ydz(i));
                        Z_DQN(h+1,2)= Z_DQN(h+1,2)+ 0.5*(-Xdz(i)*Yqn(j)+Xqz(i)*Ydn(j)-Xdz(j)*Yqn(i)+Xqz(j)*Ydn(i));              

                        Z_DQN(h+1,5)= Z_DQN(h+1,5)+ 0.5*(-Xdp(i)*Ydp(j)+Xqp(i)*Yqp(j)-Xdp(j)*Ydp(i)+Xqp(j)*Yqp(i));
                        Z_DQN(h+1,5)= Z_DQN(h+1,5)+ 0.5*(+Xdn(i)*Ydz(j)+Xqn(i)*Yqz(j)+Xdn(j)*Ydz(i)+Xqn(j)*Yqz(i)); 
                        Z_DQN(h+1,5)= Z_DQN(h+1,5)+ 0.5*(+Xdz(i)*Ydn(j)+Xqz(i)*Yqn(j)+Xdz(j)*Ydn(i)+Xqz(j)*Yqn(i));  
                    end
                end
            end
        end  
    end
    
    
    Z_DQN(1,1) =     Zdc(1);
    Z_DQN(1,2) =     Zdc(2);
    Z_DQN(1,3) =     Zdc(3);
    Z_DQN(1,4) =     Zdc(4);
    Z_DQN(1,5) =     Zdc(5);
    Z_DQN(1,6) =     Zdc(6);
    


    for i = 1 : N + HrmDbl*N + 1
     
        if(i>1)
            Zdcpnz_c(1,i) = (Z_DQN(i,1)) + 1i*Z_DQN(i,4);
            Zdcpnz_c(2,i) = (-Z_DQN(i,2)) + 1i*Z_DQN(i,5);
            Zdcpnz_c(3,i) = (Z_DQN(i,3)) + 1i*Z_DQN(i,6);
        else

            Zdcpnz_c(1,i) = 0.5*(Z_DQN(i,4) - 1i*Z_DQN(i,1));
            Zdcpnz_c(2,i) = 0.5*(Z_DQN(i,5) + 1i*Z_DQN(i,2));
            Zdcpnz_c(3,i) =     (Z_DQN(i,6) + 1i*Z_DQN(i,3));
        end
    
    end
    
end

== matlab function DQN_ABC_Test/MATLAB Function1 ==
  data: Xpnz_ci input; Xabc output; tho input; HRM parameter; Xpnz_c output
function [Xabc,Xpnz_c] = fcn(Xpnz_ci, tho, HRM)

Xabc = zeros(3,1);


a = -0.5+0.866i;
a2 = -0.5-0.866i;
Sas = [1,a,a2;1,a2,a;1,1,1]/3;
Ssa = inv(Sas);

for i = 1 : HRM+1


    if(i>1)
        h = i-1;

        th = h*tho;
    
        mag_p = abs(Xpnz_ci(1,i));
        ang_p = angle(Xpnz_ci(1,i));
        mag_n = abs(Xpnz_ci(2,i));
        ang_n = angle(Xpnz_ci(2,i));
        mag_z = abs(Xpnz_ci(3,i));
        ang_z = angle(Xpnz_ci(3,i));
        
        abc3p = mag_p*[sin(th+ang_p) ; sin(th+ang_p-2*pi/3) ; sin(th+ang_p+2*pi/3) ];
        abc3n = mag_n*[sin(th+ang_n) ; sin(th+ang_n+2*pi/3) ; sin(th+ang_n-2*pi/3) ];
        abc3z = mag_z*[sin(th+ang_z) ; sin(th+ang_z)        ; sin(th+ang_z)  ];
    
        Xabc = Xabc + abc3p+abc3n+abc3z;
    else
        Xabc = Xabc + real(Ssa*(Xpnz_ci(:,1)));
    
    end

Xpnz_c = Xpnz_ci;
    
end

== matlab function DQN_ABC_Test/ABC1/Int ==
  data: x input; z output; dt parameter
function z = fcn(x, dt)

    persistent z_old;    
    persistent x_old;   
    persistent dt2;
    
    if(isempty(dt2))
        dt2 = dt/2; 
        z_old  = zeros(3,1);
        x_old  = zeros(3,1);
    end
    
    R = 1.3;
    iL = 1000;
    Krl1 = (dt2*iL/(1+dt2*R*iL));
    Krl2 = (1-dt2*R*iL)/(1+dt2*R*iL);
    
    z = zeros(3,1);

    %z = (dt2)*(x+x_old)+z_old;
    z = Krl1*(x+x_old)+Krl2*z_old;
    z_old = z;
    x_old = x;
    
end

== matlab function DQN_ABC_Test/Int_DQN_Mat4 ==
  settings: updateMethod=DISCRETE
  data: Xpnz input; N parameter; dt parameter; w parameter; InitInt parameter; Zpnz output
function Zpnz    = Int_DQN_Mat(Xpnz, N, dt, w, InitInt)

    nrSig = 1;

    Zpnz = complex(zeros(3,N+1));

    persistent Zpnz_old;
    persistent Xpnz_old;


        dt2 = dt/2;
        
    if(isempty(Zpnz_old)) 
    
        a = -0.5+0.866i;
        a2 = -0.5-0.866i;
        Sas = [1,a,a2;1,a2,a;1,1,1]/3;
        
        Zpnz_old = complex(zeros(3,N+1));
        Xpnz_old = complex(zeros(3,N+1));
        
        if(~isempty(InitInt))
        Zpnz_old(:,1) = Sas * InitInt;
        
        end
            
    end
       
    
    for k = 1 : nrSig
    
        Zpnz(:,1) = dt2*(Xpnz(:,1)+Xpnz_old(:,1)) + Zpnz_old(:,1);

        Xpnz_old(:,1) = Xpnz(:,1);
        Zpnz_old(:,1) = Zpnz(:,1);


        if(N>0)

            for i = 1 : N
                wn =  i * w; 

                wndt2 = wn*dt2;
                A = 1/(1+(dt2*wn)^2);

                %%% POS %%%
                K1 = dt*real(Xpnz(1,i+1)) + real(Zpnz_old(1,i+1))      + imag(Zpnz_old(1,i+1))*wndt2;
                K2 = dt*imag(Xpnz(1,i+1)) -real(Zpnz_old(1,i+1))*wndt2 + imag(Zpnz_old(1,i+1));

                % Zdp(i) = (A)*( real(Xpnz(1,i+1))+imag(Zpnz_old(1,i+1))*wndt2/dt2 + real(Zpnz_old(1,i+1))*(1-wndt2^2)/2/dt2 + wndt2*imag(Xpnz(1,i+1)) );
                % Zqp(i) = (A)*( imag(Xpnz(1,i+1))-real(Zpnz_old(1,i+1))*wndt2/dt2 + imag(Zpnz_old(1,i+1))*(1-wndt2^2)/2/dt2 - wndt2*real(Xpnz(1,i+1)) );

                Zpnz(1,i+1) = A*( ( K1 + wndt2*K2) + 1i*( K2 - wndt2*K1) );

                %%% NEG %%%
                K1 = dt2*(2*real(Xpnz(2,i+1))+imag(Zpnz_old(2,i+1))*wn) + real(Zpnz_old(2,i+1));
                K2 = dt2*(2*imag(Xpnz(2,i+1))-real(Zpnz_old(2,i+1))*wn) + imag(Zpnz_old(2,i+1));

                Zpnz(2,i+1) = A*( K1 + wndt2*K2) + 1i*A*( K2 - wndt2*K1);

                %%% ZERO %%%
                K1 = dt2*(2*real(Xpnz(3,i+1))+imag(Zpnz_old(3,i+1))*wn) + real(Zpnz_old(3,i+1));
                K2 = dt2*(2*imag(Xpnz(3,i+1))-real(Zpnz_old(3,i+1))*wn) + imag(Zpnz_old(3,i+1));

                Zpnz(3,i+1) = A*( K1 + wndt2*K2) + 1i*A*( K2 - wndt2*K1);
                Zpnz_old(:,i+1) = Zpnz(:,i+1);


            end

        end

    end
end

== matlab function DQN_ABC_Test/Gain_DQNc_Mat4 ==
  data: Xpnz input; Ypnz output; Rabc parameter; chkInv parameter; HRM parameter
function Ypnz  = Gain_Mat2(Xpnz, Rabc, chkInv, HRM)
    persistent Rpnz;
    %persistent nrInp;
    persistent nrOut;

    mrows = size(Rabc,1)/3; %signal size
    mcols = size(Rabc,2)/3; %signal size

    nrInp = size(Rabc,1);

    % Ypnz = complex(zeros(nrInp, HRM+1));


    if(isempty(Rpnz)) 

        Rpnz = complex(zeros(3*mrows,3*mcols));
        a = -0.5+0.866i;
        a2 = -0.5-0.866i;
        Sas = [1,a,a2;1,a2,a;1,1,1]/3;
        %Ssa = eye(3)/(Sas);
        %nrInp = size(Xpnz,1) / 3;

        for i = 1 : mrows
            for j = 1 : mcols
                Rpnz((1:3) + (i-1)*3,(1:3) + (j-1)*3) = Sas*Rabc((1:3) + (i-1)*3,(1:3) + (j-1)*3)/Sas;
            end
        end

        if(chkInv)
            %Rpnz((1:3) + (i-1)*3,(1:3) + (j-1)*3) = eye(3)/Rpnz((1:3) + (i-1)*3,(1:3) + (j-1)*3);
            Rpnz = eye(3*mrows,3*mcols)/Rpnz;
        end

    end




    
    Ypnz = Rpnz*Xpnz;

end

== matlab function DQN_ABC_Test/Int_DQN_Mat2 ==
  settings: updateMethod=DISCRETE
  data: Z_DQN output; Xdcpnz_c input; N parameter; dt parameter; w parameter; EMT parameter; InitInt parameter; Zdcpnz_c output
function [Z_DQN, Zdcpnz_c] = Int_DQN_Mat(Xdcpnz_c, N, dt, w, EMT, InitInt)


    X_DQN = zeros(N+1,6);
    Zdcpnz_c = complex(zeros(3,N+1));

    X_DQN(1,4) =  2*real(Xdcpnz_c(1,1));
    X_DQN(1,5) =  2*real(Xdcpnz_c(2,1));
    X_DQN(1,6) =  real(Xdcpnz_c(3,1));

    X_DQN(1,1) =  -2*imag(Xdcpnz_c(1,1));
    X_DQN(1,2) =  2*imag(Xdcpnz_c(2,1));
    X_DQN(1,3) =  imag(Xdcpnz_c(3,1));

    for i = 2 : N + 1
    
        X_DQN(i,1) =  real(Xdcpnz_c(1,i));
        X_DQN(i,2) = -real(Xdcpnz_c(2,i));
        X_DQN(i,3) =  real(Xdcpnz_c(3,i));

        X_DQN(i,4) =  imag(Xdcpnz_c(1,i));
        X_DQN(i,5) =  imag(Xdcpnz_c(2,i));
        X_DQN(i,6) =  imag(Xdcpnz_c(3,i));
   
    end



    persistent Z_DQN_old;

    persistent Zdc_old;    
    persistent Xdc_old;   
    persistent Zdp_old;    
    persistent Zqp_old;    
    persistent Zdn_old;    
    persistent Zqn_old;    
    persistent Zdz_old;    
    persistent Zqz_old;  
       
    nrSig  = size(X_DQN,2)/6; 
    Z_DQN = zeros(1*N+1,6*nrSig);


    if(mod(size(X_DQN,2),6) ~= 0)
        error('Invalid input!');
    end
    
    
    for k = 1 : nrSig
    
        ok = (k-1)*6;

        Xdp = X_DQN(:,ok+1);
        Xdn = X_DQN(:,ok+2);
        Xdz = X_DQN(:,ok+3);
        Xqp = X_DQN(:,ok+4);
        Xqn = X_DQN(:,ok+5);
        Xqz = X_DQN(:,ok+6);



        dt2 = dt/2;

        Tad_p2 = (2/3)*[sin(0) sin(0-2*pi/3) sin(0+2*pi/3);  
                       cos(0) cos(0-2*pi/3) cos(0+2*pi/3);];

        Tad_z2 = (1/3)*[sin(0) sin(0) sin(0);  
                       cos(0) cos(0) cos(0);];

        Ta_dqn = [Tad_p2(1,:); Tad_p2(1,:); Tad_z2(1,:); Tad_p2(2,:); Tad_p2(2,:); Tad_z2(2,:)];

        Xdc = zeros(6,1);
        Zdc = zeros(6,1);

        Xdc(1) = Xdp(1);
        Xdc(2) = Xdn(1);
        Xdc(3) = Xdz(1);
        Xdc(4) = Xqp(1);
        Xdc(5) = Xqn(1);
        Xdc(6) = Xqz(1);


        if(isempty(Zdc_old)) 
            
            Z_DQN_old = zeros(N+1,6);
            
            if(isempty(InitInt))
                Zdc_old  = zeros(nrSig*6,1);
            else
                if(nrSig*6 == numel(InitInt))
                    Zdc_old  = InitInt'; 
                else
                    Zdc_old  = zeros(nrSig*6,1);
                end
            end
                        
        end
        if(isempty(Xdc_old)) Xdc_old  = zeros(nrSig*6,1); end

        Zdc(:) = dt2*(Xdc(:)+Xdc_old(ok+1:ok+6))+Zdc_old(ok+1:ok+6);
        Zdc_old(ok+1:ok+6) = Zdc;
        Xdc_old(ok+1:ok+6) = Xdc;


        if(N>0)

            for i = 1 : N
                wn =  i * w; 

                if(EMT)

                    wndt2 = wn*dt2;
                    A = 2/(1+(dt2*wn)^2);

                    %%% POS %%%
                    K1 = dt2*(2*real(Xdcpnz_c(1,i+1))+Z_DQN_old(i+1,4)*wn) + Z_DQN_old(i+1,1);
                    K2 = dt2*(2*imag(Xdcpnz_c(1,i+1))-Z_DQN_old(i+1,1)*wn) + Z_DQN_old(i+1,4);

                    Z_DQN(i+1,1) = A*( K1 + wndt2*K2)/2;
                    Z_DQN(i+1,4) = A*( K2 - wndt2*K1)/2;



                    %%% NEG %%%
                    K1 = dt2*(-2*real(Xdcpnz_c(2,i+1))-Z_DQN_old(i+1,5)*wn) + Z_DQN_old(i+1,2);
                    K2 = dt2*(2*imag(Xdcpnz_c(2,i+1))+Z_DQN_old(i+1,2)*wn) + Z_DQN_old(i+1,5);

                    Z_DQN(i+1,2) = A*( K1 - wndt2*K2)/2;
                    Z_DQN(i+1,5) = A*( K2 + wndt2*K1)/2;



                    %%% ZERO %%%
                    K1 = dt2*(2*real(Xdcpnz_c(3,i+1))+Z_DQN_old(i+1,6)*wn) + Z_DQN_old(i+1,3);
                    K2 = dt2*(2*imag(Xdcpnz_c(3,i+1))-Z_DQN_old(i+1,3)*wn) + Z_DQN_old(i+1,6);

                    Z_DQN(i+1,3) = A*( K1 + wndt2*K2)/2;
                    Z_DQN(i+1,6) = A*( K2 - wndt2*K1)/2;

                    Z_DQN_old = Z_DQN;

                else

                    Z_DQN(i+1,1) = (imag(Xdcpnz_c(1,i+1)))*(1/(wn));
                    Z_DQN(i+1,4) = (real(Xdcpnz_c(1,i+1)))*(-1/(wn)); 

                    Z_DQN(i+1,2) = (imag(Xdcpnz_c(2,i+1)))*(-1/(wn));
                    Z_DQN(i+1,5) = (-real(Xdcpnz_c(2,i+1)))*(1/(wn)); 

                    Z_DQN(i+1,3) = (imag(Xdcpnz_c(3,i+1)))*(1/(wn));
                    Z_DQN(i+1,6) = (real(Xdcpnz_c(3,i+1)))*(-1/(wn));

                    sT = sin(2*pi/3);
                    cT = cos(2*pi/3);

                    Zdc = Zdc-Ta_dqn*[Z_DQN(i+1,4);-sT*Z_DQN(i+1,1)+cT*Z_DQN(i+1,4);sT*Z_DQN(i+1,1)+cT*Z_DQN(i+1,4)];
                    Zdc = Zdc-Ta_dqn*[Z_DQN(i+1,5);-sT*Z_DQN(i+1,2)+cT*Z_DQN(i+1,5);sT*Z_DQN(i+1,2)+cT*Z_DQN(i+1,5)];
                    Zdc = Zdc-Ta_dqn*[Z_DQN(i+1,6); Z_DQN(i+1,6)             ;Z_DQN(i+1,6)];

                end


            end


        end


        Z_DQN(1,:) = Zdc;
    end
end

== matlab function DQN_ABC_Test/ABC2/Int ==
  data: x input; z output; dt parameter
function z = fcn(x, dt)

    persistent z_old;    
    persistent x_old;   
    persistent dt2;
    
    if(isempty(dt2))
        dt2 = dt/2; 
        z_old  = zeros(3,1);
        x_old  = zeros(3,1);
    end
    
    R = 1.3;
    iL = 1000;
    Krl1 = (dt2*iL/(1+dt2*R*iL));
    Krl2 = (1-dt2*R*iL)/(1+dt2*R*iL);
    
    z = zeros(3,1);

    %z = (dt2)*(x+x_old)+z_old;
    z = Krl1*(x+x_old)+Krl2*z_old;
    z_old = z;
    x_old = x;
    
end

== matlab function DQN_ABC_Test/Gain_DQNc_Mat5 ==
  data: Xpnz input; Ypnz output; Rabc parameter; chkInv parameter; HRM parameter
function Ypnz  = Gain_Mat2(Xpnz, Rabc, chkInv, HRM)
    persistent Rpnz;
    %persistent nrInp;
    persistent nrOut;

    mrows = size(Rabc,1)/3; %signal size
    mcols = size(Rabc,2)/3; %signal size

    nrInp = size(Rabc,1);

    % Ypnz = complex(zeros(nrInp, HRM+1));


    if(isempty(Rpnz)) 

        Rpnz = complex(zeros(3*mrows,3*mcols));
        a = -0.5+0.866i;
        a2 = -0.5-0.866i;
        Sas = [1,a,a2;1,a2,a;1,1,1]/3;
        %Ssa = eye(3)/(Sas);
        %nrInp = size(Xpnz,1) / 3;

        for i = 1 : mrows
            for j = 1 : mcols
                Rpnz((1:3) + (i-1)*3,(1:3) + (j-1)*3) = Sas*Rabc((1:3) + (i-1)*3,(1:3) + (j-1)*3)/Sas;
            end
        end

        if(chkInv)
            %Rpnz((1:3) + (i-1)*3,(1:3) + (j-1)*3) = eye(3)/Rpnz((1:3) + (i-1)*3,(1:3) + (j-1)*3);
            Rpnz = eye(3*mrows,3*mcols)/Rpnz;
        end

    end




    
    Ypnz = Rpnz*Xpnz;

end

== matlab function DQN_ABC_Test/Ihistory_Flux1/Gain_DQNc_Mat2 ==
  data: Xabc input; Ypnz output
 function Ypnz  = Gain_Mat2(Xabc)
    persistent Sas;

    if(isempty(Sas)) 
        a  = -0.5+1i*sqrt(3)/2;
        a2 = -0.5-1i*sqrt(3)/2;
        Sas = [1,a,a2;1,a2,a;1,1,1]/3;
    end
    
    Ypnz = Sas*Xabc/Sas;

end

== matlab function DQN_ABC_Test/Ihistory_Flux1/Gain_DQNc_Mat3 ==
  data: Xabc input; Ypnz output
function Ypnz  = Gain_Mat2(Xabc)
    persistent Sas;

    if(isempty(Sas)) 
        a = -0.5+0.866i;
        a2 = -0.5-0.866i;
        Sas = [1,a,a2;1,a2,a;1,1,1]/3;
    end
    
    Ypnz = Sas*Xabc/Sas;

end

== matlab function DQN_ABC_Test/Int_DQN_fdbk2/Int_d_2N_2 ==
  settings: updateMethod=DISCRETE
  data: Zdp output; Xdp input; Xdn input; Xdz input; Xqp input; Xqn input; Xqz input; Zdn output; N parameter; dt parameter; w parameter; Zdz output; Zqp output; Zqn output; Zqz output; R parameter; iL parameter; SW parameter
function [Zdp,Zdn,Zdz,Zqp,Zqn,Zqz]  = IntDQN(Xdp, Xdn, Xdz, Xqp, Xqn, Xqz, N, dt, w, R, iL, SW)

    persistent Zdc_old;    
    persistent Xdc_old;   
    persistent Zdp_old;    
    persistent Zqp_old;    
    persistent Zdn_old;    
    persistent Zqn_old;    
    persistent Zdz_old;    
    persistent Zqz_old;  
    persistent Krl1;
    persistent Krl2;
       
    persistent dt2;
    persistent range;
       
    Xdc = zeros(6,1);
    Zdc = zeros(6,1);
    
    Xdc(1) = Xdp(1);
    Xdc(2) = Xdn(1);
    Xdc(3) = Xdz(1);
    Xdc(4) = Xqp(1);
    Xdc(5) = Xqn(1);
    Xdc(6) = Xqz(1);

    Xdp = [Xdp(2:end); zeros(N-numel(Xdp)+1,1)];
    Xqp = [Xqp(2:end); zeros(N-numel(Xqp)+1,1)];
    Xdn = [Xdn(2:end); zeros(N-numel(Xdn)+1,1)];
    Xqn = [Xqn(2:end); zeros(N-numel(Xqn)+1,1)];
    Xdz = [Xdz(2:end); zeros(N-numel(Xdz)+1,1)];
    Xqz = [Xqz(2:end); zeros(N-numel(Xqz)+1,1)];
       
    Zdp = zeros(N+1,1);
    Zdn = zeros(N+1,1);
    Zqp = zeros(N+1,1);
    Zqn = zeros(N+1,1);
    Zdz = zeros(N+1,1);
    Zqz = zeros(N+1,1);
       
    if(isempty(Zdp_old)) 
        Zdc_old  = zeros(6,1); %Zdc_old  = InitInt';
        Xdc_old  = zeros(6,1);
        
        Zdp_old  = zeros(N,1);% Zdp_old(1) = InitInt(1);
        Zdn_old  = zeros(N,1);% Zdn_old(1) = InitInt(2);
        Zdz_old  = zeros(N,1);% Zdz_old(1) = InitInt(3);
        Zqp_old  = zeros(N,1);% Zqp_old(1) = InitInt(4);
        Zqn_old  = zeros(N,1);% Zqn_old(1) = InitInt(5);
        Zqz_old  = zeros(N,1);% Zqz_old(1) = InitInt(6);
        
        dt2 = dt/2;  
        range = N; 
        
        if(SW)
            Krl1 = (iL/(1+dt2*R*iL));
            Krl2 = (1-dt2*R*iL)/(1+dt2*R*iL);
        else
            Krl1 = 1;
            Krl2 = 1;
        end
        
    end

    
    
    %Zdc(:) = dt2*(Xdc(:)+Xdc_old(:))+Zdc_old(:);
    Zdc(:) = Krl1*dt2*(Xdc(:)+Xdc_old(:))+Krl2*Zdc_old(:);
    
    
    Zdc_old = Zdc;
    Xdc_old = Xdc;
    
    if(N>0)
              
        for i = 1 : range

            wn =  i * w;
            wndt2 = wn*dt2;
            A = 2*dt2/(1+wndt2^2);
            B = (1-wndt2^2)/(1+wndt2^2);

            %%% NEG %%%
            Zdp(i) = Krl1*A*(Xdp(i)+wndt2*Xqp(i))+Krl2*(B*Zdp_old(i)+A*wn*Zqp_old(i));
            Zqp(i) = Krl1*A*(Xqp(i)-wndt2*Xdp(i))+Krl2*(B*Zqp_old(i)-A*wn*Zdp_old(i));

            Zdp_old(i) = Zdp(i);
            Zqp_old(i) = Zqp(i); 


            %%% NEG %%%
            Zdn(i) = Krl1*A*(Xdn(i)-wndt2*Xqn(i))+Krl2*(B*Zdn_old(i)-A*wn*Zqn_old(i));
            Zqn(i) = Krl1*A*(Xqn(i)+wndt2*Xdn(i))+Krl2*(B*Zqn_old(i)+A*wn*Zdn_old(i));

            Zdn_old(i) = Zdn(i);
            Zqn_old(i) = Zqn(i); 

            %%% ZERO %%%
            Zdz(i) = Krl1*A*(Xdz(i)+wndt2*Xqz(i))+Krl2*(B*Zdz_old(i)+A*wn*Zqz_old(i));
            Zqz(i) = Krl1*A*(Xqz(i)-wndt2*Xdz(i))+Krl2*(B*Zqz_old(i)-A*wn*Zdz_old(i));

            Zdz_old(i) = Zdz(i);
            Zqz_old(i) = Zqz(i); 
        end

        Zdp(2:end) = Zdp(1:end-1);
        Zdn(2:end) = Zdn(1:end-1);
        Zdz(2:end) = Zdz(1:end-1);
        Zqp(2:end) = Zqp(1:end-1);
        Zqn(2:end) = Zqn(1:end-1);
        Zqz(2:end) = Zqz(1:end-1);


    end
    
    Zdp(1)     = Zdc(1);
    Zdn(1)     = Zdc(2);
    Zdz(1)     = Zdc(3);
    Zqp(1)     = Zdc(4);
    Zqn(1)     = Zdc(5);
    Zqz(1)     = Zdc(6);
end

== matlab function DQN_ABC_Test/Ihistory_Flux1/Gain_DQNc_Mat4 ==
  data: Xabc input; Ypnz output
function Ypnz  = Gain_Mat2(Xabc)
    persistent Sas;

    if(isempty(Sas)) 
        a = -0.5+0.866i;
        a2 = -0.5-0.866i;
        Sas = [1,a,a2;1,a2,a;1,1,1]/3;
    end
    
    Ypnz = Sas*Xabc/Sas;

end

== matlab function DQN_ABC_Test/Ihistory_Flux1/Gain_DQNc_Mat5 ==
  data: Xabc input; Ypnz output
function Ypnz  = Gain_Mat2(Xabc)
    persistent Sas;

    if(isempty(Sas)) 
        a = -0.5+0.866i;
        a2 = -0.5-0.866i;
        Sas = [1,a,a2;1,a2,a;1,1,1]/3;
    end
    
    Ypnz = Sas*Xabc/Sas;

end

== matlab function DQN_ABC_Test/Gain_DQNc_Mat3 ==
  data: Xpnz input; Ypnz output; Rabc parameter; chkInv parameter; HRM parameter
function Ypnz  = Gain_Mat2(Xpnz, Rabc, chkInv, HRM)
    persistent Rpnz;
    %persistent nrInp;
    persistent nrOut;

    mrows = size(Rabc,1)/3; %signal size
    mcols = size(Rabc,2)/3; %signal size

    nrInp = size(Rabc,1);

    Ypnz = complex(zeros(nrInp, HRM+1));


    if(isempty(Rpnz)) 

        Rpnz = complex(zeros(3*mrows,3*mcols));
        a = -0.5+0.866i;
        a2 = -0.5-0.866i;
        Sas = [1,a,a2;1,a2,a;1,1,1]/3;
        %Ssa = eye(3)/(Sas);
        %nrInp = size(Xpnz,1) / 3;

        for i = 1 : mrows
            for j = 1 : mcols
                oi = (i-1)*6;
                oj = (j-1)*6;
                Rpnz((1:3) + (i-1)*3,(1:3) + (j-1)*3) = Sas*Rabc((1:3) + (i-1)*3,(1:3) + (j-1)*3)/Sas;
            end
        end

        if(chkInv)
            %Rpnz((1:3) + (i-1)*3,(1:3) + (j-1)*3) = eye(3)/Rpnz((1:3) + (i-1)*3,(1:3) + (j-1)*3);
            Rpnz = eye(3*mrows,3*mcols)/Rpnz;
        end

    end




    
    Ypnz = Rpnz*Xpnz;

end

== matlab function DQN_ABC_Test/Ihistory_Flux/Gain_DQNc_Mat6 ==
  data: Xabc input; Ypnz output
 function Ypnz  = Gain_Mat2(Xabc)
    persistent Sas;

    if(isempty(Sas)) 
        a  = -0.5+1i*sqrt(3)/2;
        a2 = -0.5-1i*sqrt(3)/2;
        Sas = [1,a,a2;1,a2,a;1,1,1]/3;
    end
    
    Ypnz = Sas*Xabc/Sas;

end
